simulink model "driveTurtlebot"  (R2020b)
settings: Solver=FixedStepAuto  StartTime=0.0  StopTime=inf  RelTol=1e-3
StopFcn:
  | figHandles = findobj('Type', 'figure');
  | for i = 1: length(figHandles)
  |     if contains(figHandles(i).Name, 'Sign Following Robot', 'IgnoreCase', true)
  |         close(figHandles(i));
  |     end
  | end
  | 
  | clear figHandles;
model workspace (MAT data in the model file):
  SL_ROS_VariableLengthArrays_MaxSizes.CommonInfo.ArrayTruncateAction = 'EmitWarning'
  SL_ROS_VariableLengthArrays_MaxSizes.MsgTypeMap = containers.Map
  SL_ROS_VariableLengthArrays_MaxSizes.MsgTypeMap.serialization.keys = {'sensor_msgs/Image'}
  SL_ROS_VariableLengthArrays_MaxSizes.MsgTypeMap.serialization.values{1}(1).PropertyName = 'Data'
  SL_ROS_VariableLengthArrays_MaxSizes.MsgTypeMap.serialization.values{1}(1).DataType = 'uint8'
  SL_ROS_VariableLengthArrays_MaxSizes.MsgTypeMap.serialization.values{1}(1).MaxLength = 921600
  SL_ROS_VariableLengthArrays_MaxSizes.MsgTypeMap.serialization.values{1}(2).PropertyName = 'Encoding'
  SL_ROS_VariableLengthArrays_MaxSizes.MsgTypeMap.serialization.values{1}(2).DataType = 'uint8'
  SL_ROS_VariableLengthArrays_MaxSizes.MsgTypeMap.serialization.values{1}(2).MaxLength = 128
  SL_ROS_VariableLengthArrays_MaxSizes.MsgTypeMap.serialization.uniformity = 0
  SL_ROS_VariableLengthArrays_MaxSizes.MsgTypeMap.serialization.keyType = 'char'
  SL_ROS_VariableLengthArrays_MaxSizes.MsgTypeMap.serialization.valueType = 'any'
undefined symbols (not defined in the file): Angular, Linear
libraries: robotlib x2
settings Model: Creator=The MathWorks, Inc.  LastModifiedBy=josea
settings OptimizationCC: EnhancedBackFolding=on  PassReuseOutputArgsThreshold=0  MaxStackSize=64  OptimizeBlockOrder=speed  DifferentSizesBufferReuse=on  OptimizationCustomize=off
settings DebuggingCC: ParameterTunabilityLossMsg=error
settings HardwareCC: ProdBitPerPointer=32  ProdBitPerSizeT=32  ProdBitPerPtrDiffT=32  ProdLargestAtomicFloat=None  ProdIntDivRoundTo=Undefined  ProdEndianess=Unspecified  ProdWordSize=32  ProdHWDeviceType=Generic->Unspecified (assume 32-bit Generic)  UseEmbeddedCoderFeatures=off
settings SFSimCC: MATLABDynamicMemAlloc=off  SimTargetLang=C++
settings RTWCC: Description=Embedded Coder  SystemTargetFile=ert.tlc  HardwareBoard=Robot Operating System (ROS)  TLCOptions="-aInlineSetEventsForThisBaseRateFcn=TLC_FALSE -aSuppressMultiTaskScheduler=TLC_FALSE  -aRateBasedStepFcn=0"  TemplateMakefile=ert_default_tmf  GenerateReport=on  Toolchain=Catkin  LaunchReport=on  TargetLang=C++
settings CodeAppCC: ForceParamTrailComments=on  OperatorAnnotations=on
settings ERTTargetCC: ERTCustomFileBanners=off  SupportContinuousTime=on  SupportNonInlinedSFcns=on  RemoveResetFunc=off  SupportVariableSizeSignals=on  ModelStepFunctionPrototypeControlCompliant=off

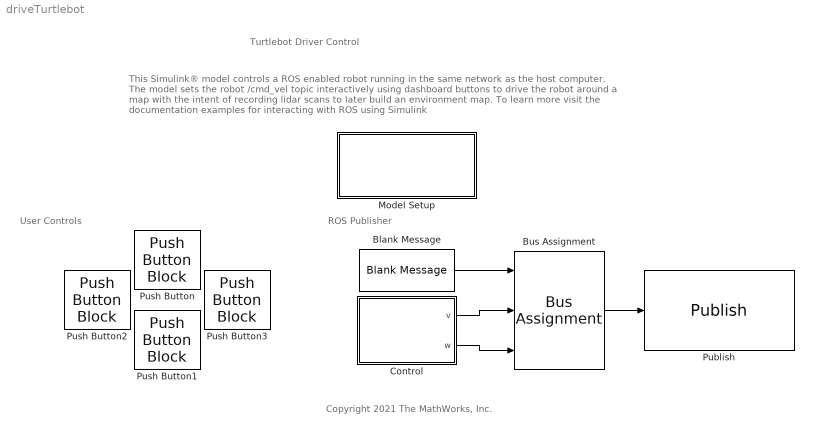
== system driveTurtlebot ==
  note: This Simulink® model controls a ROS enabled robot running in the same network as the host computer. The model sets the robot /cmd_vel topic interactively using dashboard buttons to drive the robot around a map with the intent of recording lidar scans to later build an environment map. To learn more visit the documentation examples for interacting with ROS using Simulink
  note: Turtlebot Driver Control
  note: ROS Publisher
  note: User Controls
  note: Copyright 2021 The MathWorks, Inc.
  Blank Message : robotlib/Blank Message  messageClass=Message  entityType=geometry_msgs/Twist  messageType=geometry_msgs/Twist  SampleTime=inf  legacyBusStruct=off
  Bus Assignment : BusAssignment  AssignedSignals=Linear.X,Angular.Z
  Control : Subsystem
  Model Setup : Subsystem
  Publish : robotlib/Publish  topicSource=Select from ROS network  topic=/cmd_vel  messageType=geometry_msgs/Twist  legacyBusStruct=off  messageQueueLength=1
  Push Button : PushButtonBlock  ButtonText=Fwd
  Push Button1 : PushButtonBlock  ButtonText=Rev  OnValue=-1
  Push Button2 : PushButtonBlock  ButtonText=Left
  Push Button3 : PushButtonBlock  ButtonText=Right  OnValue=-1
  wires:
  Bus Assignment/1 -> Publish/1
  Blank Message/1 -> Bus Assignment/1
  Control/1(v) -> Bus Assignment/2
  Control/2(w) -> Bus Assignment/3

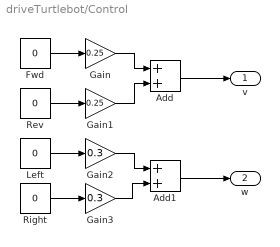
== system driveTurtlebot/Control ==
  Add : Sum
  Add1 : Sum
  Fwd : Constant  Value=0
  Gain : Gain  Gain=0.25
  Gain1 : Gain  Gain=0.25
  Gain2 : Gain  Gain=0.3
  Gain3 : Gain  Gain=0.3
  Left : Constant  Value=0
  Rev : Constant  Value=0
  Right : Constant  Value=0
  v : Outport
  w : Outport  Port=2
  wires:
  Rev/1 -> Gain1/1
  Add/1 -> v/1
  Left/1 -> Gain2/1
  Fwd/1 -> Gain/1
  Right/1 -> Gain3/1
  Add1/1 -> w/1
  Gain/1 -> Add/1
  Gain1/1 -> Add/2
  Gain2/1 -> Add1/1
  Gain3/1 -> Add1/2

== system driveTurtlebot/Model Setup ==
  note: Before running the Simulink model, make sure the ROS network requirements have been set appropriately through the Simulink Toolstrip. Note that setting a Node Host IP address is optional and depends on the computer setup.
  note: ROS Model Setup
